simulink model "IEEE30_case"  (R2024b)
settings: Solver=FixedStepAuto  StartTime=0  StopTime=5  FixedStep=1e-7  RelTol=1e-3
values from neighbouring files (symbols this model uses):
  GFL_DFIG_7_C_bus = 0.08    [IEEE30_case_parameters.m]
  GFL_DFIG_7_D_mutual = 2.500000e+3    (= 2500)    [IEEE30_case_parameters.m]
  GFL_DFIG_7_f0 = 60    [IEEE30_case_parameters.m]
  GFL_DFIG_7_gPLLi = 3200    [IEEE30_case_parameters.m]
  GFL_DFIG_7_gPLLp = 650    [IEEE30_case_parameters.m]
  GFL_DFIG_7_H_WT = 0.4    [IEEE30_case_parameters.m]
  GFL_DFIG_7_Hg = 0.8    [IEEE30_case_parameters.m]
  GFL_DFIG_7_Igq_ref = 0    [IEEE30_case_parameters.m]
  GFL_DFIG_7_Ird_ref = 704.45696    [IEEE30_case_parameters.m]
  GFL_DFIG_7_KI_V = -300000    [IEEE30_case_parameters.m]
  GFL_DFIG_7_KP_V = -1000    [IEEE30_case_parameters.m]
  GFL_DFIG_7_Ksh = 1.254300e+4    (= 12543)    [IEEE30_case_parameters.m]
  GFL_DFIG_7_Lg = 0.000483    [IEEE30_case_parameters.m]
  GFL_DFIG_7_Lm_pu = 4    [IEEE30_case_parameters.m]
  GFL_DFIG_7_N = 100    [IEEE30_case_parameters.m]
  GFL_DFIG_7_p = 2    [IEEE30_case_parameters.m]
  GFL_DFIG_7_Pitch = 0    [IEEE30_case_parameters.m]
  GFL_DFIG_7_R = 44    [IEEE30_case_parameters.m]
  GFL_DFIG_7_Rg = 2.000000e-5    (= 2e-05)    [IEEE30_case_parameters.m]
  GFL_DFIG_7_rho = 1.225    [IEEE30_case_parameters.m]
  GFL_DFIG_7_rPLLi = 4500    [IEEE30_case_parameters.m]
  GFL_DFIG_7_rPLLp = 620    [IEEE30_case_parameters.m]
  GFL_DFIG_7_Rs_pu = 0.011    [IEEE30_case_parameters.m]
  GFL_DFIG_7_Sbase = 2.000000e+6    (= 2000000)    [IEEE30_case_parameters.m]
  GFL_DFIG_7_ugq_ref = 0    [IEEE30_case_parameters.m]
  GFL_DFIG_7_usd_ref = 0    [IEEE30_case_parameters.m]
  GFL_DFIG_7_Vbase = 690    [IEEE30_case_parameters.m]
  GFL_DFIG_7_Vdc_ref = 1200    [IEEE30_case_parameters.m]
  GFL_DFIG_7_wind = 12    [IEEE30_case_parameters.m]
  GFL_DFIG_7_wm_ref = 518.184209    [IEEE30_case_parameters.m]
  SG_D_13_D = 0.01056    [IEEE30_case_parameters.m]
  SG_D_13_EnableSaturation = 0    [IEEE30_case_parameters.m]
  SG_D_13_f0 = 60    [IEEE30_case_parameters.m]
  SG_D_13_H = 7.5    [IEEE30_case_parameters.m]
  SG_D_13_K_A = 20    [IEEE30_case_parameters.m]
  SG_D_13_K_E = 1.000000e+1    (= 10)    [IEEE30_case_parameters.m]
  SG_D_13_K_F = 2.363    [IEEE30_case_parameters.m]
  SG_D_13_K_s = 0.5    [IEEE30_case_parameters.m]
  SG_D_13_R_a = 0.001088    [IEEE30_case_parameters.m]
  SG_D_13_S_A = 1    [IEEE30_case_parameters.m]
  SG_D_13_S_B = 0.103    [IEEE30_case_parameters.m]
  SG_D_13_S_N = 10.659857    [IEEE30_case_parameters.m]
  SG_D_13_SpeedPara = 200    [IEEE30_case_parameters.m]
  SG_D_13_T_0 = 0.370163    [IEEE30_case_parameters.m]
  SG_D_13_T_1 = 0.3    [IEEE30_case_parameters.m]
  SG_D_13_T_2 = 0.05    [IEEE30_case_parameters.m]
  SG_D_13_T_3 = 0.02    [IEEE30_case_parameters.m]
  SG_D_13_T_4 = 0.005    [IEEE30_case_parameters.m]
  SG_D_13_T_A = 0.02    [IEEE30_case_parameters.m]
  SG_D_13_T_dd = 8.000000e+0    (= 8)    [IEEE30_case_parameters.m]
  SG_D_13_T_ddd = 0.04    [IEEE30_case_parameters.m]
  SG_D_13_T_E = 0.314    [IEEE30_case_parameters.m]
  SG_D_13_T_F = 0.35    [IEEE30_case_parameters.m]
  SG_D_13_T_qd = 0.8    [IEEE30_case_parameters.m]
  SG_D_13_T_qdd = 0.02    [IEEE30_case_parameters.m]
  SG_D_13_T_speed = 0.1    [IEEE30_case_parameters.m]
  SG_D_13_T_w = 0.5    [IEEE30_case_parameters.m]
  SG_D_13_V_ref = 1.696619    [IEEE30_case_parameters.m]
  SG_D_13_w_ref = 376.991118    [IEEE30_case_parameters.m]
  SG_D_13_x_d = 1.9    [IEEE30_case_parameters.m]
  SG_D_13_x_dd = 0.302    [IEEE30_case_parameters.m]
  SG_D_13_x_ddd = 0.204    [IEEE30_case_parameters.m]
  SG_D_13_x_l = 0.05    [IEEE30_case_parameters.m]
  SG_D_13_x_q = 1.3    [IEEE30_case_parameters.m]
  SG_D_13_x_qd = 0.5    [IEEE30_case_parameters.m]
  SG_D_13_x_qdd = 0.3    [IEEE30_case_parameters.m]
  SG_D_1_D = 0.01056    [IEEE30_case_parameters.m]
  SG_D_1_EnableSaturation = 0    [IEEE30_case_parameters.m]
  SG_D_1_f0 = 60    [IEEE30_case_parameters.m]
  SG_D_1_H = 7.5    [IEEE30_case_parameters.m]
  SG_D_1_K_A = 20    [IEEE30_case_parameters.m]
  SG_D_1_K_E = 1.000000e+1    (= 10)    [IEEE30_case_parameters.m]
  SG_D_1_K_F = 2.363    [IEEE30_case_parameters.m]
  SG_D_1_K_s = 0.5    [IEEE30_case_parameters.m]
  SG_D_1_R_a = 0.001088    [IEEE30_case_parameters.m]
  SG_D_1_S_A = 1    [IEEE30_case_parameters.m]
  SG_D_1_S_B = 0.103    [IEEE30_case_parameters.m]
  SG_D_1_S_N = 10.659857    [IEEE30_case_parameters.m]
  SG_D_1_SpeedPara = 200    [IEEE30_case_parameters.m]
  SG_D_1_T_0 = 0.259812    [IEEE30_case_parameters.m]
  SG_D_1_T_1 = 0.3    [IEEE30_case_parameters.m]
  SG_D_1_T_2 = 0.05    [IEEE30_case_parameters.m]
  SG_D_1_T_3 = 0.02    [IEEE30_case_parameters.m]
  SG_D_1_T_4 = 0.005    [IEEE30_case_parameters.m]
  SG_D_1_T_A = 0.02    [IEEE30_case_parameters.m]
  SG_D_1_T_dd = 8.000000e+0    (= 8)    [IEEE30_case_parameters.m]
  SG_D_1_T_ddd = 0.04    [IEEE30_case_parameters.m]
  SG_D_1_T_E = 0.314    [IEEE30_case_parameters.m]
  SG_D_1_T_F = 0.35    [IEEE30_case_parameters.m]
  SG_D_1_T_qd = 0.8    [IEEE30_case_parameters.m]
  SG_D_1_T_qdd = 0.02    [IEEE30_case_parameters.m]
  SG_D_1_T_speed = 0.1    [IEEE30_case_parameters.m]
  SG_D_1_T_w = 0.5    [IEEE30_case_parameters.m]
  SG_D_1_V_ref = 1.544107    [IEEE30_case_parameters.m]
  SG_D_1_w_ref = 376.991118    [IEEE30_case_parameters.m]
  SG_D_1_x_d = 1.9    [IEEE30_case_parameters.m]
  SG_D_1_x_dd = 0.302    [IEEE30_case_parameters.m]
  SG_D_1_x_ddd = 0.204    [IEEE30_case_parameters.m]
  SG_D_1_x_l = 0.05    [IEEE30_case_parameters.m]
  SG_D_1_x_q = 1.3    [IEEE30_case_parameters.m]
  SG_D_1_x_qd = 0.5    [IEEE30_case_parameters.m]
  SG_D_1_x_qdd = 0.3    [IEEE30_case_parameters.m]
  SG_D_22_D = 0.01056    [IEEE30_case_parameters.m]
  SG_D_22_EnableSaturation = 0    [IEEE30_case_parameters.m]
  SG_D_22_f0 = 60    [IEEE30_case_parameters.m]
  SG_D_22_H = 7.5    [IEEE30_case_parameters.m]
  SG_D_22_K_A = 20    [IEEE30_case_parameters.m]
  SG_D_22_K_E = 1.000000e+1    (= 10)    [IEEE30_case_parameters.m]
  SG_D_22_K_F = 2.363    [IEEE30_case_parameters.m]
  SG_D_22_K_s = 0.5    [IEEE30_case_parameters.m]
  SG_D_22_R_a = 0.001088    [IEEE30_case_parameters.m]
  SG_D_22_S_A = 1    [IEEE30_case_parameters.m]
  SG_D_22_S_B = 0.103    [IEEE30_case_parameters.m]
  SG_D_22_S_N = 10.659857    [IEEE30_case_parameters.m]
  SG_D_22_SpeedPara = 200    [IEEE30_case_parameters.m]
  SG_D_22_T_0 = 0.216121    [IEEE30_case_parameters.m]
  SG_D_22_T_1 = 0.3    [IEEE30_case_parameters.m]
  SG_D_22_T_2 = 0.05    [IEEE30_case_parameters.m]
  SG_D_22_T_3 = 0.02    [IEEE30_case_parameters.m]
  SG_D_22_T_4 = 0.005    [IEEE30_case_parameters.m]
  ... (+126 more)
(part 12 of 27)

== system IEEE30_case/GFL_DFIG_7/d_Phi_gb_GFL_DFIG_7_block ==
  note: d_Phi_gb_GFL_DFIG_7 in IEEE30_case
      | $-4\,\mathrm{Lg}\,{f_{0}}^2\,\pi ^2\,\left(i_{\mathrm{gd},\mathrm{GFL},\mathrm{DFIG},7}-\frac{0.666666666666667\,\Phi _{\mathrm{gc},\mathrm{GFL},\mathrm{DFIG},7}-0.666666666666667\,\mathrm{KP}_{V}\,\left(V_{\mathrm{dc},\mathrm{GFL},\mathrm{DFIG},7}-\mathrm{Vdc}_{\mathrm{ref}}\right)}{\mathrm{Vbase}}\right)$
      | Automatically generated on 2025-11-01 18:34:05 .
  State_i_gd_GFL_DFIG_7_640f4 : Inport
  State_V_dc_GFL_DFIG_7_6d222 : Inport  Port=2
  State_Phi_gc_GFL_DFIG_7_b7107 : Inport  Port=3
  Add_6bffb : Sum
  Add_b5257 : Sum
  Add_b8cf5 : Sum
  Constant_-1_6b980 : Constant  Value=-1
  Constant_-1_cf33c : Constant  Value=-1
  Constant_0.666666666666667_f141c : Constant  Value=0.666666666666667
  Constant_2.0_6b877 : Constant  Value=2.0
  Constant_2.0_f717f : Constant  Value=2.0
  Constant_4.0_b6ef0 : Constant  Value=4.0
  Constant_KP_V_1bd51 : Constant  Value=KP_V
  Constant_Lg_6a87d : Constant  Value=Lg
  Constant_Vbase_73b54 : Constant  Value=Vbase
  Constant_Vdc_ref_f08aa : Constant  Value=Vdc_ref
  Constant_f0_de8e9 : Constant  Value=f0
  Constant_pi_e3308 : Constant  Value=pi
  Divide_9162a : Product  Inputs=*/
  Power_585c5 : Math  Operator=pow
  Power_96685 : Math  Operator=pow
  Product_0199e : Product
  Product_1d506 : Product
  Product_26373 : Product
  Product_b2acb : Product
  Product_c600a : Product
  Product_cfa46 : Product
  Product_d4dd0 : Product
  Product_f39e3 : Product
  Blockout_d_Phi_gb_GFL_DFIG_7_12bfd : Outport
  wires:
  Constant_-1_6b980/1 -> Product_d4dd0/1
  Constant_Vdc_ref_f08aa/1 -> Add_b8cf5/2
  Constant_pi_e3308/1 -> Power_96685/1
  Constant_Vbase_73b54/1 -> Divide_9162a/2
  Add_b8cf5/1 -> Product_c600a/2
  State_V_dc_GFL_DFIG_7_6d222/1 -> Product_d4dd0/2
  Product_d4dd0/1 -> Add_b8cf5/1
  State_i_gd_GFL_DFIG_7_640f4/1 -> Product_1d506/2
  Constant_KP_V_1bd51/1 -> Product_c600a/1
  Constant_2.0_f717f/1 -> Power_96685/2
  Product_c600a/1 -> Add_b5257/1
  State_Phi_gc_GFL_DFIG_7_b7107/1 -> Add_b5257/2
  Constant_4.0_b6ef0/1 -> Product_26373/1
  Power_96685/1 -> Product_26373/2
  Constant_0.666666666666667_f141c/1 -> Product_cfa46/1
  Product_0199e/1 -> Product_b2acb/1
  Add_b5257/1 -> Product_cfa46/2
  Product_26373/1 -> Product_f39e3/1
  Constant_f0_de8e9/1 -> Power_585c5/1
  Constant_Lg_6a87d/1 -> Product_f39e3/2
  Constant_2.0_6b877/1 -> Power_585c5/2
  Constant_-1_cf33c/1 -> Product_1d506/1
  Product_cfa46/1 -> Divide_9162a/1
  Product_f39e3/1 -> Product_0199e/1
  Power_585c5/1 -> Product_0199e/2
  Product_1d506/1 -> Add_6bffb/1
  Divide_9162a/1 -> Add_6bffb/2
  Add_6bffb/1 -> Product_b2acb/2
  Product_b2acb/1 -> Blockout_d_Phi_gb_GFL_DFIG_7_12bfd/1

== system IEEE30_case/GFL_DFIG_7/d_Phi_gc_GFL_DFIG_7_block ==
  note: d_Phi_gc_GFL_DFIG_7 in IEEE30_case
      | $-\mathrm{KI}_{V}\,\left(V_{\mathrm{dc},\mathrm{GFL},\mathrm{DFIG},7}-\mathrm{Vdc}_{\mathrm{ref}}\right)$
      | Automatically generated on 2025-11-01 18:34:03 .
  State_V_dc_GFL_DFIG_7_30c65 : Inport
  Add_e8db4 : Sum
  Constant_-1_5cb89 : Constant  Value=-1
  Constant_KI_V_c5ac4 : Constant  Value=KI_V
  Constant_Vdc_ref_57ce9 : Constant  Value=Vdc_ref
  Product_3b29a : Product
  Product_b79c6 : Product
  Blockout_d_Phi_gc_GFL_DFIG_7_e7a32 : Outport
  wires:
  Constant_-1_5cb89/1 -> Product_3b29a/1
  State_V_dc_GFL_DFIG_7_30c65/1 -> Product_3b29a/2
  Product_3b29a/1 -> Add_e8db4/1
  Product_b79c6/1 -> Blockout_d_Phi_gc_GFL_DFIG_7_e7a32/1
  Constant_Vdc_ref_57ce9/1 -> Add_e8db4/2
  Constant_KI_V_c5ac4/1 -> Product_b79c6/1
  Add_e8db4/1 -> Product_b79c6/2

== system IEEE30_case/GFL_DFIG_7/d_Phi_ra_GFL_DFIG_7_block ==
  note: d_Phi_ra_GFL_DFIG_7 in IEEE30_case
      | $\frac{121.601990049751\,\pi \,{\mathrm{Rs}_{\mathrm{pu}}}^2\,{\mathrm{Vbase}}^2\,f_{0}\,\left(\mathrm{Ird}_{\mathrm{ref}}-\frac{100.497512437811\,\pi \,\Psi _{\mathrm{dr},\mathrm{GFL},\mathrm{DFIG},7}\,\mathrm{Sbase}\,f_{0}}{\mathrm{Lm}_{\mathrm{pu}}\,{\mathrm{Vbase}}^2}+\frac{99.502487562189\,\pi \,\Psi _{\mathrm{ds},\mathrm{GFL},\mathrm{DFIG},7}\,\mathrm{Sbase}\,f_{0}}{\mathrm{Lm}_{\mathrm{pu}}\,{\mathrm{Vbase}}^2}\right)}{\mathrm{Lm}_{\mathrm{pu}}\,\mathrm{Sbase}}$
      | Automatically generated on 2025-11-01 18:33:11 .
  State_Psi_dr_GFL_DFIG_7_3e6d6 : Inport
  State_Psi_ds_GFL_DFIG_7_9adb5 : Inport  Port=2
  Add_f4b53 : Sum
  Constant_100.497512437811_3d4e5 : Constant  Value=100.497512437811
  Constant_121.601990049751_8103e : Constant  Value=121.601990049751
  Constant_2.0_5d4a4 : Constant  Value=2.0
  Constant_2.0_83c42 : Constant  Value=2.0
  Constant_2.0_893ba : Constant  Value=2.0
  Constant_2.0_ddf2f : Constant  Value=2.0
  Constant_99.502487562189_4b56a : Constant  Value=99.502487562189
  Constant_Ird_ref_83d74 : Constant  Value=Ird_ref
  Constant_Lm_pu_11795 : Constant  Value=Lm_pu
  Constant_Lm_pu_a81e2 : Constant  Value=Lm_pu
  Constant_Lm_pu_dbc9c : Constant  Value=Lm_pu
  Constant_Rs_pu_66a36 : Constant  Value=Rs_pu
  Constant_Sbase_aa7f6 : Constant  Value=Sbase
  Constant_Sbase_e8890 : Constant  Value=Sbase
  Constant_Sbase_efa73 : Constant  Value=Sbase
  Constant_Vbase_4a93a : Constant  Value=Vbase
  Constant_Vbase_63b23 : Constant  Value=Vbase
  Constant_Vbase_ff58f : Constant  Value=Vbase
  Constant_f0_6d6a3 : Constant  Value=f0
  Constant_f0_798e9 : Constant  Value=f0
  Constant_f0_b0c51 : Constant  Value=f0
  Constant_pi_37fdb : Constant  Value=pi
  Constant_pi_c8d94 : Constant  Value=pi
  Constant_pi_e7969 : Constant  Value=pi
  Divide_0905f : Product  Inputs=*/
  Divide_383a0 : Product  Inputs=*/
  Divide_99316 : Product  Inputs=*/
  Power_35857 : Math  Operator=pow
  Power_5b5c9 : Math  Operator=pow
  Power_dc40c : Math  Operator=pow
  Power_df89a : Math  Operator=pow
  Product_081b4 : Product
  Product_09a91 : Product
  Product_12e3f : Product
  Product_15670 : Product
  Product_186d4 : Product
  Product_26318 : Product
  Product_38ada : Product
  Product_3f361 : Product
  Product_5c4f4 : Product
  Product_684e9 : Product
  Product_8995b : Product
  Product_96f38 : Product
  Product_aa582 : Product
  Product_b7735 : Product
  Product_d9359 : Product
  Product_d9bcd : Product
  Subtract_8a7b5 : Sum  Inputs=+-
  Blockout_d_Phi_ra_GFL_DFIG_7_b9bb2 : Outport
  wires:
  Constant_Sbase_efa73/1 -> Product_12e3f/2
  Constant_100.497512437811_3d4e5/1 -> Product_38ada/1
  Constant_Vbase_ff58f/1 -> Power_5b5c9/1
  Product_96f38/1 -> Product_15670/1
  Constant_2.0_83c42/1 -> Power_35857/2
  Constant_pi_37fdb/1 -> Product_38ada/2
  State_Psi_dr_GFL_DFIG_7_3e6d6/1 -> Product_96f38/2
  Product_d9bcd/1 -> Product_5c4f4/1
  Product_38ada/1 -> Product_96f38/1
  Constant_99.502487562189_4b56a/1 -> Product_26318/1
  Product_5c4f4/1 -> Product_186d4/1
  Constant_pi_c8d94/1 -> Product_26318/2
  Constant_Vbase_63b23/1 -> Power_dc40c/1
  Constant_Sbase_aa7f6/1 -> Product_15670/2
  Constant_Vbase_4a93a/1 -> Power_df89a/1
  Constant_2.0_893ba/1 -> Power_df89a/2
  Product_26318/1 -> Product_aa582/1
  State_Psi_ds_GFL_DFIG_7_9adb5/1 -> Product_aa582/2
  Constant_Sbase_e8890/1 -> Product_8995b/2
  Constant_Rs_pu_66a36/1 -> Power_35857/1
  Constant_121.601990049751_8103e/1 -> Product_d9bcd/1
  Constant_pi_e7969/1 -> Product_d9bcd/2
  Product_8995b/1 -> Divide_99316/2
  Product_15670/1 -> Product_081b4/1
  Product_3f361/1 -> Product_b7735/1
  Constant_f0_798e9/1 -> Product_081b4/2
  Product_b7735/1 -> Divide_99316/1
  Constant_Lm_pu_a81e2/1 -> Product_684e9/1
  Power_df89a/1 -> Product_684e9/2
  Product_aa582/1 -> Product_12e3f/1
  Constant_2.0_5d4a4/1 -> Power_5b5c9/2
  Power_35857/1 -> Product_5c4f4/2
  Constant_2.0_ddf2f/1 -> Power_dc40c/2
  Product_081b4/1 -> Divide_0905f/1
  Product_684e9/1 -> Divide_0905f/2
  Product_12e3f/1 -> Product_09a91/1
  Divide_383a0/1 -> Add_f4b53/2
  Constant_f0_6d6a3/1 -> Product_09a91/2
  Constant_Lm_pu_11795/1 -> Product_d9359/1
  Power_5b5c9/1 -> Product_d9359/2
  Power_dc40c/1 -> Product_186d4/2
  Constant_Ird_ref_83d74/1 -> Subtract_8a7b5/1
  Divide_0905f/1 -> Subtract_8a7b5/2
  Product_09a91/1 -> Divide_383a0/1
  Product_d9359/1 -> Divide_383a0/2
  Product_186d4/1 -> Product_3f361/1
  Constant_f0_b0c51/1 -> Product_3f361/2
  Subtract_8a7b5/1 -> Add_f4b53/1
  Add_f4b53/1 -> Product_b7735/2
  Constant_Lm_pu_dbc9c/1 -> Product_8995b/1
  Divide_99316/1 -> Blockout_d_Phi_ra_GFL_DFIG_7_b9bb2/1

== system IEEE30_case/GFL_DFIG_7/d_Phi_rb_GFL_DFIG_7_block ==
  note: d_Phi_rb_GFL_DFIG_7 in IEEE30_case
      | $-\frac{121.601990049751\,\pi \,{\mathrm{Rs}_{\mathrm{pu}}}^2\,{\mathrm{Vbase}}^2\,f_{0}\,\left(\frac{0.673333333333333\,\Phi _{\mathrm{rc},\mathrm{GFL},\mathrm{DFIG},7}-\frac{10.773333333333328\,\mathrm{Sbase}\,p\,\left(w_{m,\mathrm{GFL},\mathrm{DFIG},7}-\mathrm{wm}_{\mathrm{ref}}\right)}{{f_{0}}^2\,\pi ^2}}{p\,\sqrt{{\Psi _{\mathrm{ds},\mathrm{GFL},\mathrm{DFIG},7}}^2+{\Psi _{\mathrm{qs},\mathrm{GFL},\mathrm{DFIG},7}}^2}}+\frac{100.497512437811\,\pi \,\Psi _{\mathrm{qr},\mathrm{GFL},\mathrm{DFIG},7}\,\mathrm{Sbase}\,f_{0}}{\mathrm{Lm}_{\mathrm{pu}}\,{\mathrm{Vbase}}^2}-\frac{99.502487562189\,\pi \,\Psi _{\mathrm{qs},\mathrm{GFL},\mathrm{DFIG},7}\,\mathrm{Sbase}\,f_{0}}{\mathrm{Lm}_{\mathrm{pu}}\,{\mathrm{Vbase}}^2}\right)}{\mathrm{Lm}_{\mathrm{pu}}\,\mathrm{Sbase}}$
      | Automatically generated on 2025-11-01 18:33:17 .
  State_Phi_rc_GFL_DFIG_7_bc2c9 : Inport
  State_w_m_GFL_DFIG_7_5425d : Inport  Port=2
  State_Psi_ds_GFL_DFIG_7_7a16b : Inport  Port=3
  State_Psi_qs_GFL_DFIG_7_57503 : Inport  Port=4
  State_Psi_qr_GFL_DFIG_7_e4388 : Inport  Port=5
  State_Psi_qs_GFL_DFIG_7_e35cc : Inport  Port=6
  Add_8c335 : Sum
  Add_8e695 : Sum
  Add_9cf97 : Sum
  Add_d9e26 : Sum
  Constant_-0.673333333333333_fade5 : Constant  Value=-0.673333333333333
  Constant_-1_8d982 : Constant  Value=-1
  Constant_100.497512437811_2b07e : Constant  Value=100.497512437811
  Constant_121.601990049751_b651a : Constant  Value=121.601990049751
  Constant_16.0_b18cb : Constant  Value=16.0
  Constant_2.0_154d8 : Constant  Value=2.0
  Constant_2.0_24e66 : Constant  Value=2.0
  Constant_2.0_2b9f3 : Constant  Value=2.0
  Constant_2.0_3bf41 : Constant  Value=2.0
  Constant_2.0_59165 : Constant  Value=2.0
  Constant_2.0_c1799 : Constant  Value=2.0
  Constant_2.0_c26f1 : Constant  Value=2.0
  Constant_2.0_f645a : Constant  Value=2.0
  Constant_99.502487562189_3da1b : Constant  Value=99.502487562189
  Constant_Lm_pu_c3cbe : Constant  Value=Lm_pu
  Constant_Lm_pu_c51f7 : Constant  Value=Lm_pu
  Constant_Lm_pu_fef3e : Constant  Value=Lm_pu
  Constant_Rs_pu_8b800 : Constant  Value=Rs_pu
  Constant_Sbase_1934d : Constant  Value=Sbase
  Constant_Sbase_2886b : Constant  Value=Sbase
  Constant_Sbase_44824 : Constant  Value=Sbase
  Constant_Sbase_acc82 : Constant  Value=Sbase
  Constant_Vbase_057c8 : Constant  Value=Vbase
  Constant_Vbase_33be2 : Constant  Value=Vbase
  Constant_Vbase_c886f : Constant  Value=Vbase
  Constant_f0_37fb8 : Constant  Value=f0
  Constant_f0_64fd6 : Constant  Value=f0
  Constant_f0_d2cee : Constant  Value=f0
  Constant_f0_e037e : Constant  Value=f0
  Constant_p_9dc95 : Constant  Value=p
  Constant_p_ae0c5 : Constant  Value=p
  Constant_pi_2d1cb : Constant  Value=pi
  Constant_pi_5eceb : Constant  Value=pi
  Constant_pi_5ef27 : Constant  Value=pi
  Constant_pi_b22d2 : Constant  Value=pi
  Constant_wm_ref_5b7e7 : Constant  Value=wm_ref
  Divide_0adfc : Product  Inputs=*/
  Divide_2d540 : Product  Inputs=*/
  Divide_6bab9 : Product  Inputs=*/
  Divide_9109e : Product  Inputs=*/
  Divide_a367a : Product  Inputs=*/
  MathFunc_sqrt_aa524 : Sqrt
  Power_02213 : Math  Operator=pow
  Power_34a99 : Math  Operator=pow
  Power_4517e : Math  Operator=pow
  Power_abf73 : Math  Operator=pow
  Power_c1057 : Math  Operator=pow
  Power_c8651 : Math  Operator=pow
  Power_d591f : Math  Operator=pow
  Power_f198e : Math  Operator=pow
  Product_105da : Product
  Product_147e3 : Product
  Product_24720 : Product
  Product_307a1 : Product
  Product_3f565 : Product
  Product_436c9 : Product
  Product_4cf24 : Product
  Product_5f731 : Product
  Product_6572c : Product
  Product_6d301 : Product
  Product_6da22 : Product
  Product_6ecc6 : Product
  Product_96586 : Product
  Product_99f2d : Product
  Product_a3501 : Product
  Product_ba56f : Product
  Product_c0d1a : Product
  Product_c2194 : Product
  Product_c2604 : Product
  Product_d5eee : Product
  Product_dfcd2 : Product
  Product_e7fe8 : Product
  Product_eb59e : Product
  Subtract_2b91f : Sum  Inputs=+-
  Blockout_d_Phi_rb_GFL_DFIG_7_7ae6c : Outport
  wires:
  Constant_Sbase_acc82/1 -> Product_96586/2
  Constant_16.0_b18cb/1 -> Product_dfcd2/1
  Constant_p_9dc95/1 -> Product_6da22/2
  Product_5f731/1 -> Divide_0adfc/1
  State_Psi_qr_GFL_DFIG_7_e4388/1 -> Product_a3501/2
  Constant_Sbase_2886b/1 -> Product_dfcd2/2
  Constant_100.497512437811_2b07e/1 -> Product_147e3/1
  Constant_wm_ref_5b7e7/1 -> Add_9cf97/2
  Constant_Lm_pu_c51f7/1 -> Product_99f2d/1
  Constant_-1_8d982/1 -> Product_c2604/1
  Product_dfcd2/1 -> Product_6da22/1
  State_w_m_GFL_DFIG_7_5425d/1 -> Product_c2604/2
  Product_99f2d/1 -> Divide_2d540/2
  Product_c2604/1 -> Add_9cf97/1
  Constant_pi_b22d2/1 -> Power_4517e/1
  Constant_2.0_c1799/1 -> Power_4517e/2
  Product_c2194/1 -> Product_105da/1
  Constant_f0_64fd6/1 -> Power_f198e/1
  Constant_2.0_2b9f3/1 -> Power_f198e/2
  Product_147e3/1 -> Product_a3501/1
  Product_6da22/1 -> Product_6ecc6/1
  Add_9cf97/1 -> Product_6ecc6/2
  Power_4517e/1 -> Product_eb59e/1
  Product_105da/1 -> Product_6572c/1
  Product_3f565/1 -> Product_ba56f/1
  Power_f198e/1 -> Product_eb59e/2
  State_Psi_ds_GFL_DFIG_7_7a16b/1 -> Power_34a99/1
  Constant_2.0_c26f1/1 -> Power_34a99/2
  State_Psi_qs_GFL_DFIG_7_57503/1 -> Power_02213/1
  Constant_2.0_f645a/1 -> Power_02213/2
  Constant_pi_2d1cb/1 -> Product_147e3/2
  Product_a3501/1 -> Product_96586/1
  Product_6ecc6/1 -> Divide_9109e/1
  Product_eb59e/1 -> Divide_9109e/2
  Constant_pi_5eceb/1 -> Product_3f565/2
  Power_34a99/1 -> Add_8e695/1
  Constant_2.0_3bf41/1 -> Power_c8651/2
  Power_02213/1 -> Add_8e695/2
  Power_abf73/1 -> Product_ba56f/2
  Constant_99.502487562189_3da1b/1 -> Product_d5eee/1
  Constant_pi_5ef27/1 -> Product_d5eee/2
  State_Phi_rc_GFL_DFIG_7_bc2c9/1 -> Add_d9e26/1
  Product_96586/1 -> Product_6d301/1
  Divide_9109e/1 -> Add_d9e26/2
  Constant_Vbase_33be2/1 -> Power_d591f/1
  Add_8e695/1 -> MathFunc_sqrt_aa524/1
  Constant_Vbase_057c8/1 -> Power_c1057/1
  Constant_2.0_154d8/1 -> Power_c1057/2
  Product_d5eee/1 -> Product_c2194/1
  State_Psi_qs_GFL_DFIG_7_e35cc/1 -> Product_c2194/2
  Constant_121.601990049751_b651a/1 -> Product_3f565/1
  Constant_Sbase_1934d/1 -> Product_105da/2
  Constant_Rs_pu_8b800/1 -> Power_abf73/1
  Product_4cf24/1 -> Divide_6bab9/2
  Constant_2.0_24e66/1 -> Power_abf73/2
  Constant_-0.673333333333333_fade5/1 -> Product_307a1/1
  Add_d9e26/1 -> Product_307a1/2
  Constant_p_ae0c5/1 -> Product_4cf24/1
  MathFunc_sqrt_aa524/1 -> Product_4cf24/2
  Constant_f0_d2cee/1 -> Product_6d301/2
  Power_c1057/1 -> Product_99f2d/2
  Constant_Vbase_c886f/1 -> Power_c8651/1
  Constant_2.0_59165/1 -> Power_d591f/2
  Product_307a1/1 -> Divide_6bab9/1
  Product_6d301/1 -> Divide_2d540/1
  Constant_f0_e037e/1 -> Product_6572c/2
  Constant_Lm_pu_c3cbe/1 -> Product_c0d1a/1
  Power_c8651/1 -> Product_c0d1a/2
  Product_ba56f/1 -> Product_436c9/1
  Power_d591f/1 -> Product_436c9/2
  Divide_6bab9/1 -> Subtract_2b91f/1
  Divide_2d540/1 -> Subtract_2b91f/2
  Product_6572c/1 -> Divide_a367a/1
  Product_c0d1a/1 -> Divide_a367a/2
  Product_436c9/1 -> Product_24720/1
  Constant_f0_37fb8/1 -> Product_24720/2
  Subtract_2b91f/1 -> Add_8c335/1
  Divide_a367a/1 -> Add_8c335/2
  Product_24720/1 -> Product_5f731/1
  Add_8c335/1 -> Product_5f731/2
  Constant_Lm_pu_fef3e/1 -> Product_e7fe8/1
  Constant_Sbase_44824/1 -> Product_e7fe8/2
  Product_e7fe8/1 -> Divide_0adfc/2
  Divide_0adfc/1 -> Blockout_d_Phi_rb_GFL_DFIG_7_7ae6c/1

== system IEEE30_case/GFL_DFIG_7/d_Phi_rc_GFL_DFIG_7_block ==
  note: d_Phi_rc_GFL_DFIG_7 in IEEE30_case
      | $-\frac{128\,\mathrm{Sbase}\,p\,\left(w_{m,\mathrm{GFL},\mathrm{DFIG},7}-\mathrm{wm}_{\mathrm{ref}}\right)}{\mathrm{Hg}\,{f_{0}}^2\,\pi ^2}$
      | Automatically generated on 2025-11-01 18:33:13 .
  State_w_m_GFL_DFIG_7_b5946 : Inport
  Add_033cf : Sum
  Constant_-1_a203c : Constant  Value=-1
  Constant_128.0_a6df2 : Constant  Value=128.0
  Constant_2.0_1c071 : Constant  Value=2.0
  Constant_2.0_c935a : Constant  Value=2.0
  Constant_Hg_01f24 : Constant  Value=Hg
  Constant_Sbase_867f4 : Constant  Value=Sbase
  Constant_f0_a5d67 : Constant  Value=f0
  Constant_p_14ae6 : Constant  Value=p
  Constant_pi_9f808 : Constant  Value=pi
  Constant_wm_ref_67022 : Constant  Value=wm_ref
  Divide_7ffd1 : Product  Inputs=*/
  Power_0f740 : Math  Operator=pow
  Power_99261 : Math  Operator=pow
  Product_167f3 : Product
  Product_23ecd : Product
  Product_336df : Product
  Product_343c6 : Product
  Product_bafc2 : Product
  Product_d8355 : Product
  Blockout_d_Phi_rc_GFL_DFIG_7_aa447 : Outport
  wires:
  Constant_p_14ae6/1 -> Product_167f3/2
  Constant_128.0_a6df2/1 -> Product_343c6/1
  State_w_m_GFL_DFIG_7_b5946/1 -> Product_23ecd/2
  Constant_Sbase_867f4/1 -> Product_343c6/2
  Product_bafc2/1 -> Divide_7ffd1/1
  Constant_2.0_c935a/1 -> Power_99261/2
  Constant_-1_a203c/1 -> Product_23ecd/1
  Constant_Hg_01f24/1 -> Product_336df/2
  Product_23ecd/1 -> Add_033cf/1
  Constant_pi_9f808/1 -> Power_99261/1
  Product_343c6/1 -> Product_167f3/1
  Constant_wm_ref_67022/1 -> Add_033cf/2
  Power_99261/1 -> Product_336df/1
  Constant_f0_a5d67/1 -> Power_0f740/1
  Add_033cf/1 -> Product_bafc2/2
  Constant_2.0_1c071/1 -> Power_0f740/2
  Product_167f3/1 -> Product_bafc2/1
  Product_336df/1 -> Product_d8355/1
  Power_0f740/1 -> Product_d8355/2
  Product_d8355/1 -> Divide_7ffd1/2
  Divide_7ffd1/1 -> Blockout_d_Phi_rc_GFL_DFIG_7_aa447/1

== system IEEE30_case/GFL_DFIG_7/d_Phipllg_GFL_DFIG_7_block ==
  note: d_Phipllg_GFL_DFIG_7 in IEEE30_case
      | $-\mathrm{gPLLi}\,\left(\mathrm{ugq}_{\mathrm{ref}}+v_{q,\mathrm{GFL},\mathrm{DFIG},7}\,\cos\left(\theta _{\mathrm{pllg},\mathrm{GFL},\mathrm{DFIG},7}\right)+v_{d,\mathrm{GFL},\mathrm{DFIG},7}\,\sin\left(\theta _{\mathrm{pllg},\mathrm{GFL},\mathrm{DFIG},7}\right)\right)$
      | Automatically generated on 2025-11-01 18:34:08 .
  Input_v_d_GFL_DFIG_7_9bb07 : Inport
  State_theta_pllg_GFL_DFIG_7_d7c88 : Inport  Port=2
  Input_v_q_GFL_DFIG_7_4b381 : Inport  Port=3
  State_theta_pllg_GFL_DFIG_7_1f5b3 : Inport  Port=4
  Constant_-1_a8696 : Constant  Value=-1
  Constant_gPLLi_864bf : Constant  Value=gPLLi
  Constant_ugq_ref_056c0 : Constant  Value=ugq_ref
  MathFunc_cos_0cf31 : Trigonometry  Operator=cos
  MathFunc_sin_67054 : Trigonometry
  Product_3b1f1 : Product
  Product_a74be : Product
  Product_b0d09 : Product
  Product_c8c10 : Product
  Subtract_e5638 : Sum  Inputs=+-
  Subtract_ead05 : Sum  Inputs=+-
  Blockout_d_Phipllg_GFL_DFIG_7_57d75 : Outport
  wires:
  State_theta_pllg_GFL_DFIG_7_d7c88/1 -> MathFunc_sin_67054/1
  MathFunc_sin_67054/1 -> Product_3b1f1/2
  Constant_-1_a8696/1 -> Product_c8c10/1
  Input_v_d_GFL_DFIG_7_9bb07/1 -> Product_3b1f1/1
  Constant_ugq_ref_056c0/1 -> Product_c8c10/2
  State_theta_pllg_GFL_DFIG_7_1f5b3/1 -> MathFunc_cos_0cf31/1
  Product_c8c10/1 -> Subtract_ead05/1
  Product_3b1f1/1 -> Subtract_ead05/2
  Input_v_q_GFL_DFIG_7_4b381/1 -> Product_b0d09/1
  MathFunc_cos_0cf31/1 -> Product_b0d09/2
  Subtract_ead05/1 -> Subtract_e5638/1
  Constant_gPLLi_864bf/1 -> Product_a74be/1
  Product_b0d09/1 -> Subtract_e5638/2
  Subtract_e5638/1 -> Product_a74be/2
  Product_a74be/1 -> Blockout_d_Phipllg_GFL_DFIG_7_57d75/1

== system IEEE30_case/GFL_DFIG_7/d_Phipllr_GFL_DFIG_7_block ==
  note: d_Phipllr_GFL_DFIG_7 in IEEE30_case
      | $-\mathrm{rPLLi}\,\left(\mathrm{usd}_{\mathrm{ref}}+v_{d,\mathrm{GFL},\mathrm{DFIG},7}\,\cos\left(\theta _{\mathrm{pllr},\mathrm{GFL},\mathrm{DFIG},7}\right)-v_{q,\mathrm{GFL},\mathrm{DFIG},7}\,\sin\left(\theta _{\mathrm{pllr},\mathrm{GFL},\mathrm{DFIG},7}\right)\right)$
      | Automatically generated on 2025-11-01 18:34:06 .
  Input_v_d_GFL_DFIG_7_0a8be : Inport
  State_theta_pllr_GFL_DFIG_7_673d7 : Inport  Port=2
  Input_v_q_GFL_DFIG_7_661f6 : Inport  Port=3
  State_theta_pllr_GFL_DFIG_7_c3596 : Inport  Port=4
  Add_40468 : Sum
  Constant_-1_1c422 : Constant  Value=-1
  Constant_rPLLi_c38ff : Constant  Value=rPLLi
  Constant_usd_ref_0a1f3 : Constant  Value=usd_ref
  MathFunc_cos_0c009 : Trigonometry  Operator=cos
  MathFunc_sin_3ef5a : Trigonometry
  Product_1f9ff : Product
  Product_79bb6 : Product
  Product_8a815 : Product
  Product_fc47b : Product
  Subtract_51d6e : Sum  Inputs=+-
  Blockout_d_Phipllr_GFL_DFIG_7_3fa24 : Outport
  wires:
  State_theta_pllr_GFL_DFIG_7_673d7/1 -> MathFunc_cos_0c009/1
  Product_8a815/1 -> Subtract_51d6e/2
  MathFunc_cos_0c009/1 -> Product_8a815/2
  Add_40468/1 -> Product_79bb6/2
  Constant_-1_1c422/1 -> Product_fc47b/1
  Product_fc47b/1 -> Subtract_51d6e/1
  Constant_usd_ref_0a1f3/1 -> Product_fc47b/2
  Input_v_d_GFL_DFIG_7_0a8be/1 -> Product_8a815/1
  State_theta_pllr_GFL_DFIG_7_c3596/1 -> MathFunc_sin_3ef5a/1
  Input_v_q_GFL_DFIG_7_661f6/1 -> Product_1f9ff/1
  MathFunc_sin_3ef5a/1 -> Product_1f9ff/2
  Subtract_51d6e/1 -> Add_40468/1
  Product_1f9ff/1 -> Add_40468/2
  Constant_rPLLi_c38ff/1 -> Product_79bb6/1
  Product_79bb6/1 -> Blockout_d_Phipllr_GFL_DFIG_7_3fa24/1

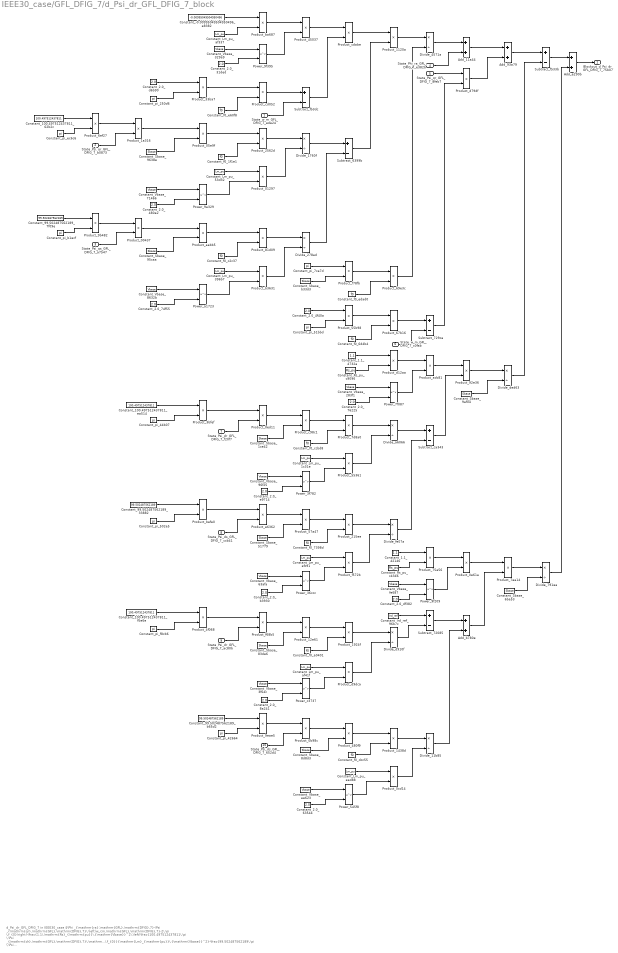
== system IEEE30_case/GFL_DFIG_7/d_Psi_dr_GFL_DFIG_7_block ==
  note: d_Psi_dr_GFL_DFIG_7 in IEEE30_case
      | $\Phi _{\mathrm{ra},\mathrm{GFL},\mathrm{DFIG},7}-\Psi _{\mathrm{qr},\mathrm{GFL},\mathrm{DFIG},7}\,\left(w_{m,\mathrm{GFL},\mathrm{DFIG},7}-2\,\pi \,f_{0}\right)-\frac{1.1\,\mathrm{Rs}_{\mathrm{pu}}\,{\mathrm{Vbase}}^2\,\left(\frac{100.497512437811\,\pi \,\Psi _{\mathrm{dr},\mathrm{GFL},\mathrm{DFIG},7}\,\mathrm{Sbase}\,f_{0}}{\mathrm{Lm}_{\mathrm{pu}}\,{\mathrm{Vbase}}^2}-\frac{99.502487562189\,\pi \,\Psi _{\mathrm{ds},\mathrm{GFL},\mathrm{DFIG},7}\,\mathrm{Sbase}\,f_{0}}{\mathrm{Lm}_{\mathrm{pu}}\,{\mathrm{Vbase}}^2}\right)}{\mathrm{Sbase}}+\frac{1.1\,\mathrm{Rs}_{\mathrm{pu}}\,{\mathrm{Vbase}}^2\,\left(\mathrm{Ird}_{\mathrm{ref}}-\frac{100.497512437811\,\pi \,\Psi _{\mathrm{dr},\mathrm{GFL},\mathrm{DFIG},7}\,\mathrm{Sbase}\,f_{0}}{\mathrm{Lm}_{\mathrm{pu}}\,{\mathrm{Vbase}}^2}+\frac{99.502487562189\,\pi \,\Psi _{\mathrm{ds},\mathrm{GFL},\mathrm{DFIG},7}\,\mathrm{Sbase}\,f_{0}}{\mathrm{Lm}_{\mathrm{pu}}\,{\mathrm{Vbase}}^2}\right)}{\mathrm{Sbase}}+\frac{0.00995049504950496\,\mathrm{Lm}_{\mathrm{pu}}\,{\mathrm{Vbase}}^2\,\left(\frac{100.497512437811\,\pi \,\Psi _{\mathrm{qr},\mathrm{GFL},\mathrm{DFIG},7}\,\mathrm{Sbase}\,f_{0}}{\mathrm{Lm}_{\mathrm{pu}}\,{\mathrm{Vbase}}^2}-\frac{99.502487562189\,\pi \,\Psi _{\mathrm{qs},\mathrm{GFL},\mathrm{DFIG},7}\,\mathrm{Sbase}\,f_{0}}{\mathrm{Lm}_{\mathrm{pu}}\,{\mathrm{Vbase}}^2}\right)\,\left(w_{m,\mathrm{GFL},\mathrm{DFIG},7}-2\,\pi \,f_{0}\right)}{\mathrm{Sbase}\,f_{0}\,\pi }$
      | Automatically generated on 2025-11-01 18:32:46 .
  State_w_m_GFL_DFIG_7_ede24 : Inport
  State_Psi_qr_GFL_DFIG_7_b0873 : Inport  Port=2
  State_Psi_qs_GFL_DFIG_7_a7547 : Inport  Port=3
  State_Phi_ra_GFL_DFIG_7_e382b : Inport  Port=4
  State_Psi_qr_GFL_DFIG_7_8feb7 : Inport  Port=5
  State_w_m_GFL_DFIG_7_c0fab : Inport  Port=6
  State_Psi_dr_GFL_DFIG_7_f20f7 : Inport  Port=7
  State_Psi_ds_GFL_DFIG_7_ccb41 : Inport  Port=8
  State_Psi_dr_GFL_DFIG_7_ac80b : Inport  Port=9
  State_Psi_ds_GFL_DFIG_7_652d4 : Inport  Port=10
  Add_11a44 : Sum
  Add_93a79 : Sum
  Add_b780e : Sum
  Add_e290b : Sum
  Constant_-0.00995049504950496_e8382 : Constant  Value=-0.00995049504950496
  Constant_1.1_42146 : Constant  Value=1.1
  Constant_1.1_4732a : Constant  Value=1.1
  Constant_100.497512437811_62b2c : Constant  Value=100.497512437811
  Constant_100.497512437811_ea514 : Constant  Value=100.497512437811
  Constant_100.497512437811_f5e6e : Constant  Value=100.497512437811
  Constant_2.0_31ded : Constant  Value=2.0
  Constant_2.0_480a2 : Constant  Value=2.0
  Constant_2.0_4f40a : Constant  Value=2.0
  Constant_2.0_63544 : Constant  Value=2.0
  Constant_2.0_74f55 : Constant  Value=2.0
  Constant_2.0_76225 : Constant  Value=2.0
  Constant_2.0_8a241 : Constant  Value=2.0
  Constant_2.0_b3930 : Constant  Value=2.0
  Constant_2.0_d6b90 : Constant  Value=2.0
  Constant_2.0_df382 : Constant  Value=2.0
  Constant_2.0_e9714 : Constant  Value=2.0
  Constant_99.502487562189_33882 : Constant  Value=99.502487562189
  Constant_99.502487562189_7f09e : Constant  Value=99.502487562189
  Constant_99.502487562189_b65d2 : Constant  Value=99.502487562189
  Constant_Ird_ref_96b7c : Constant  Value=Ird_ref
  Constant_Lm_pu_1c31e : Constant  Value=Lm_pu
  Constant_Lm_pu_396b7 : Constant  Value=Lm_pu
  Constant_Lm_pu_53d32 : Constant  Value=Lm_pu
  Constant_Lm_pu_af337 : Constant  Value=Lm_pu
  Constant_Lm_pu_af41f : Constant  Value=Lm_pu
  Constant_Lm_pu_ead88 : Constant  Value=Lm_pu
  Constant_Lm_pu_efc91 : Constant  Value=Lm_pu
  Constant_Rs_pu_c4346 : Constant  Value=Rs_pu
  Constant_Rs_pu_c9096 : Constant  Value=Rs_pu
  Constant_Sbase_1ce42 : Constant  Value=Sbase
  Constant_Sbase_51779 : Constant  Value=Sbase
  Constant_Sbase_6ba53 : Constant  Value=Sbase
  Constant_Sbase_83de6 : Constant  Value=Sbase
  Constant_Sbase_8d8d3 : Constant  Value=Sbase
  Constant_Sbase_95caa : Constant  Value=Sbase
  Constant_Sbase_9638e : Constant  Value=Sbase
  Constant_Sbase_9af04 : Constant  Value=Sbase
  Constant_Sbase_b33d3 : Constant  Value=Sbase
  Constant_Vbase_283f1 : Constant  Value=Vbase
  Constant_Vbase_329a9 : Constant  Value=Vbase
  Constant_Vbase_3f64c : Constant  Value=Vbase
  Constant_Vbase_63afa : Constant  Value=Vbase
  Constant_Vbase_71466 : Constant  Value=Vbase
  Constant_Vbase_8632b : Constant  Value=Vbase
  Constant_Vbase_96f25 : Constant  Value=Vbase
  Constant_Vbase_ae623 : Constant  Value=Vbase
  Constant_Vbase_fe687 : Constant  Value=Vbase
  Constant_f0_1f1e1 : Constant  Value=f0
  Constant_f0_6d4b4 : Constant  Value=f0
  Constant_f0_7398d : Constant  Value=f0
  Constant_f0_a0401 : Constant  Value=f0
  Constant_f0_c2c37 : Constant  Value=f0
  Constant_f0_ccbd8 : Constant  Value=f0
  Constant_f0_dcc55 : Constant  Value=f0
  Constant_f0_e60f8 : Constant  Value=f0
  Constant_f0_edad0 : Constant  Value=f0
  Constant_pi_250d6 : Constant  Value=pi
  Constant_pi_42664 : Constant  Value=pi
  Constant_pi_44b07 : Constant  Value=pi
  Constant_pi_502e5 : Constant  Value=pi
  Constant_pi_51bbd : Constant  Value=pi
  Constant_pi_7ca7d : Constant  Value=pi
  Constant_pi_b1ecf : Constant  Value=pi
  Constant_pi_ec6c6 : Constant  Value=pi
  Constant_pi_f8cb6 : Constant  Value=pi
  Divide_11b85 : Product  Inputs=*/
  Divide_1760f : Product  Inputs=*/
  Divide_278ad : Product  Inputs=*/
  Divide_4571a : Product  Inputs=*/
  Divide_791ea : Product  Inputs=*/
  Divide_a6066 : Product  Inputs=*/
  Divide_d910f : Product  Inputs=*/
  Divide_ded63 : Product  Inputs=*/
  Divide_fe07a : Product  Inputs=*/
  Power_36ccc : Math  Operator=pow
  Power_3f782 : Math  Operator=pow
  Power_545f8 : Math  Operator=pow
  Power_7f087 : Math  Operator=pow
  Power_9a329 : Math  Operator=pow
  Power_9f209 : Math  Operator=pow
  Power_9f395 : Math  Operator=pow
  Power_a1723 : Math  Operator=pow
  Power_c3737 : Math  Operator=pow
  Product_00437 : Product
  Product_01297 : Product
  Product_05e9f : Product
  Product_0b98c : Product
  Product_0cd14 : Product
  Product_0e61a : Product
  Product_0ed11 : Product
  Product_1120a : Product
  Product_12e61 : Product
  Product_1438d : Product
  Product_1924f : Product
  Product_1a316 : Product
  Product_215ee : Product
  Product_2562d : Product
  Product_33ba7 : Product
  Product_3bfef : Product
  Product_45037 : Product
  Product_480f9 : Product
  Product_4f068 : Product
  Product_55361 : Product
  Product_55b98 : Product
  Product_57a47 : Product
  Product_67b16 : Product
  Product_69e3c : Product
  Product_6ef27 : Product
  Product_75a56 : Product
  Product_7d8a0 : Product
  Product_7ea14 : Product
  Product_81d09 : Product
  Product_92e36 : Product
  Product_9b482 : Product
  Product_9eae5 : Product
  Product_aabb5 : Product
  Product_adc81 : Product
  Product_b3631 : Product
  Product_ba687 : Product
  Product_befe0 : Product
  Product_c98c1 : Product
  Product_cd052 : Product
  Product_cdabe : Product
  Product_d12aa : Product
  Product_d79df : Product
  Product_d9dca : Product
  Product_e6362 : Product
  Product_f572b : Product
  Product_f68b5 : Product
  Product_f78fb : Product
  Subtract_6399b : Sum  Inputs=+-
  Subtract_72085 : Sum  Inputs=+-
  Subtract_729ca : Sum  Inputs=+-
  Subtract_ca343 : Sum  Inputs=+-
  Subtract_f533b : Sum  Inputs=+-
  Subtract_fb3dc : Sum  Inputs=+-
  Blockout_d_Psi_dr_GFL_DFIG_7_75b07 : Outport
  wires:
  Constant_Lm_pu_efc91/1 -> Product_f572b/1
  Product_7d8a0/1 -> Divide_a6066/1
  Constant_2.0_63544/1 -> Power_545f8/2
  Constant_Sbase_6ba53/1 -> Divide_791ea/2
  Add_e290b/1 -> Blockout_d_Psi_dr_GFL_DFIG_7_75b07/1
  Constant_Vbase_3f64c/1 -> Power_c3737/1
  Subtract_ca343/1 -> Product_92e36/2
  Power_545f8/1 -> Product_0cd14/2
  State_Psi_ds_GFL_DFIG_7_652d4/1 -> Product_0b98c/2
  Product_92e36/1 -> Divide_ded63/1
  Product_81d09/1 -> Divide_278ad/1
  Constant_pi_f8cb6/1 -> Product_4f068/2
  Divide_4571a/1 -> Add_11a44/1
  Product_9eae5/1 -> Product_0b98c/1
  Constant_Lm_pu_af337/1 -> Product_ba687/2
  Constant_2.0_31ded/1 -> Power_9f395/2
  Product_01297/1 -> Divide_1760f/2
  Add_b780e/1 -> Product_7ea14/2
  Subtract_6399b/1 -> Product_1120a/2
  Product_4f068/1 -> Product_f68b5/1
  Product_0b98c/1 -> Product_480f9/1
  Product_d79df/1 -> Add_93a79/2
  State_Psi_dr_GFL_DFIG_7_ac80b/1 -> Product_f68b5/2
  Divide_791ea/1 -> Add_e290b/2
  Product_f78fb/1 -> Product_69e3c/1
  Constant_99.502487562189_b65d2/1 -> Product_9eae5/1
  Constant_pi_42664/1 -> Product_9eae5/2
  Product_adc81/1 -> Product_92e36/1
  Product_7ea14/1 -> Divide_791ea/1
  Power_7f087/1 -> Product_adc81/2
  Power_36ccc/1 -> Product_f572b/2
  Divide_11b85/1 -> Add_b780e/2
  Product_0cd14/1 -> Divide_11b85/2
  Constant_Vbase_ae623/1 -> Power_545f8/1
  Product_480f9/1 -> Product_1438d/1
  Constant_Lm_pu_ead88/1 -> Product_0cd14/1
  State_Psi_ds_GFL_DFIG_7_ccb41/1 -> Product_e6362/2
  Constant_Vbase_63afa/1 -> Power_36ccc/1
  Constant_-0.00995049504950496_e8382/1 -> Product_ba687/1
  Product_1438d/1 -> Divide_11b85/1
  Constant_100.497512437811_ea514/1 -> Product_3bfef/1
  Product_0e61a/1 -> Product_7ea14/1
  Constant_f0_c2c37/1 -> Product_81d09/2
  Constant_f0_dcc55/1 -> Product_1438d/2
  Constant_Vbase_8632b/1 -> Power_a1723/1
  Divide_ded63/1 -> Subtract_f533b/2
  Constant_Sbase_8d8d3/1 -> Product_480f9/2
  Product_f572b/1 -> Divide_fe07a/2
  Divide_d910f/1 -> Subtract_72085/2
  Product_1924f/1 -> Divide_d910f/1
  Constant_Vbase_96f25/1 -> Power_3f782/1
  Subtract_72085/1 -> Add_b780e/1
  Product_55b98/1 -> Product_67b16/1
  Subtract_f533b/1 -> Add_e290b/1
  Product_215ee/1 -> Divide_fe07a/1
  Power_a1723/1 -> Product_b3631/2
  Constant_100.497512437811_f5e6e/1 -> Product_4f068/1
  Constant_Sbase_9af04/1 -> Divide_ded63/2
  Product_d9dca/1 -> Divide_d910f/2
  Product_f68b5/1 -> Product_12e61/1
  Power_c3737/1 -> Product_d9dca/2
  Constant_Vbase_283f1/1 -> Power_7f087/1
  Constant_Ird_ref_96b7c/1 -> Subtract_72085/1
  Constant_Rs_pu_c4346/1 -> Product_75a56/2
  Constant_2.0_8a241/1 -> Power_c3737/2
  Constant_Lm_pu_af41f/1 -> Product_d9dca/1
  Product_75a56/1 -> Product_0e61a/1
  Constant_f0_a0401/1 -> Product_1924f/2
  Product_12e61/1 -> Product_1924f/1
  Constant_Sbase_83de6/1 -> Product_12e61/2
  Constant_2.0_df382/1 -> Power_9f209/2
  Constant_f0_ccbd8/1 -> Product_7d8a0/2
  Product_e6362/1 -> Product_57a47/1
  Power_9f209/1 -> Product_0e61a/2
  Constant_Vbase_fe687/1 -> Power_9f209/1
  Subtract_fb3dc/1 -> Product_cdabe/2
  Constant_1.1_42146/1 -> Product_75a56/1
  Constant_f0_7398d/1 -> Product_215ee/2
  Divide_fe07a/1 -> Subtract_ca343/2
  Constant_2.0_b3930/1 -> Power_36ccc/2
  Product_57a47/1 -> Product_215ee/1
  Constant_Sbase_51779/1 -> Product_57a47/2
  Product_befe0/1 -> Product_e6362/1
  Constant_pi_502e5/1 -> Product_befe0/2
  Constant_99.502487562189_33882/1 -> Product_befe0/1
  Divide_a6066/1 -> Subtract_ca343/1
  Product_55361/1 -> Divide_a6066/2
  Power_3f782/1 -> Product_55361/2
  Constant_2.0_e9714/1 -> Power_3f782/2
  Constant_Lm_pu_1c31e/1 -> Product_55361/1
  Product_c98c1/1 -> Product_7d8a0/1
  Constant_Sbase_1ce42/1 -> Product_c98c1/2
  Product_0ed11/1 -> Product_c98c1/1
  State_Psi_dr_GFL_DFIG_7_f20f7/1 -> Product_0ed11/2
  Product_3bfef/1 -> Product_0ed11/1
  Product_00437/1 -> Product_aabb5/1
  Constant_pi_44b07/1 -> Product_3bfef/2
  Constant_2.0_76225/1 -> Power_7f087/2
  Product_d12aa/1 -> Product_adc81/1
  Constant_Rs_pu_c9096/1 -> Product_d12aa/2
  State_w_m_GFL_DFIG_7_c0fab/1 -> Subtract_729ca/2
  Constant_1.1_4732a/1 -> Product_d12aa/1
  Add_93a79/1 -> Subtract_f533b/1
  Subtract_729ca/1 -> Product_d79df/2
  Product_67b16/1 -> Subtract_729ca/1
  Constant_f0_6d4b4/1 -> Product_67b16/2
  Constant_pi_51bbd/1 -> Product_55b98/2
  Constant_2.0_4f40a/1 -> Product_55b98/1
  State_Psi_qr_GFL_DFIG_7_8feb7/1 -> Product_d79df/1
  Add_11a44/1 -> Add_93a79/1
  State_Phi_ra_GFL_DFIG_7_e382b/1 -> Add_11a44/2
  Product_69e3c/1 -> Divide_4571a/2
  Constant_f0_edad0/1 -> Product_69e3c/2
  Constant_Sbase_b33d3/1 -> Product_f78fb/2
  Product_9b482/1 -> Product_00437/1
  Constant_pi_7ca7d/1 -> Product_f78fb/1
  Product_1120a/1 -> Divide_4571a/1
  Divide_278ad/1 -> Subtract_6399b/2
  Product_b3631/1 -> Divide_278ad/2
  Constant_2.0_74f55/1 -> Power_a1723/2
  Constant_Lm_pu_396b7/1 -> Product_b3631/1
  Product_aabb5/1 -> Product_81d09/1
  Constant_Sbase_95caa/1 -> Product_aabb5/2
  State_Psi_qs_GFL_DFIG_7_a7547/1 -> Product_00437/2
  Constant_pi_b1ecf/1 -> Product_9b482/2
  Constant_99.502487562189_7f09e/1 -> Product_9b482/1
  Divide_1760f/1 -> Subtract_6399b/1
  Power_9a329/1 -> Product_01297/2
  Constant_2.0_480a2/1 -> Power_9a329/2
  Product_2562d/1 -> Divide_1760f/1
  Constant_Vbase_71466/1 -> Power_9a329/1
  Product_45037/1 -> Product_cdabe/1
  Constant_Lm_pu_53d32/1 -> Product_01297/1
  Constant_2.0_d6b90/1 -> Product_33ba7/1
  Constant_f0_1f1e1/1 -> Product_2562d/2
  Product_05e9f/1 -> Product_2562d/1
  Constant_Sbase_9638e/1 -> Product_05e9f/2
  Product_1a316/1 -> Product_05e9f/1
  State_Psi_qr_GFL_DFIG_7_b0873/1 -> Product_1a316/2
  Product_6ef27/1 -> Product_1a316/1
  Constant_pi_ec6c6/1 -> Product_6ef27/2
  Constant_100.497512437811_62b2c/1 -> Product_6ef27/1
  Product_cdabe/1 -> Product_1120a/1
  State_w_m_GFL_DFIG_7_ede24/1 -> Subtract_fb3dc/2
  Product_cd052/1 -> Subtract_fb3dc/1
  Constant_f0_e60f8/1 -> Product_cd052/2
  Product_33ba7/1 -> Product_cd052/1
  Constant_pi_250d6/1 -> Product_33ba7/2
  Power_9f395/1 -> Product_45037/2
  Constant_Vbase_329a9/1 -> Power_9f395/1
  Product_ba687/1 -> Product_45037/1

== system IEEE30_case/GFL_DFIG_7/d_Psi_ds_GFL_DFIG_7_block ==
  note: d_Psi_ds_GFL_DFIG_7 in IEEE30_case
      | $2\,\pi \,\Psi _{\mathrm{qs},\mathrm{GFL},\mathrm{DFIG},7}\,f_{0}-\mathrm{Vbase}\,\left(v_{d,\mathrm{GFL},\mathrm{DFIG},7}\,\cos\left(\theta _{\mathrm{pllr},\mathrm{GFL},\mathrm{DFIG},7}\right)-v_{q,\mathrm{GFL},\mathrm{DFIG},7}\,\sin\left(\theta _{\mathrm{pllr},\mathrm{GFL},\mathrm{DFIG},7}\right)\right)+\frac{\mathrm{Rs}_{\mathrm{pu}}\,{\mathrm{Vbase}}^2\,\left(\frac{99.502487562189\,\pi \,\Psi _{\mathrm{dr},\mathrm{GFL},\mathrm{DFIG},7}\,\mathrm{Sbase}\,f_{0}}{\mathrm{Lm}_{\mathrm{pu}}\,{\mathrm{Vbase}}^2}-\frac{100.497512437811\,\pi \,\Psi _{\mathrm{ds},\mathrm{GFL},\mathrm{DFIG},7}\,\mathrm{Sbase}\,f_{0}}{\mathrm{Lm}_{\mathrm{pu}}\,{\mathrm{Vbase}}^2}\right)}{\mathrm{Sbase}}$
      | Automatically generated on 2025-11-01 18:32:31 .
  State_Psi_qs_GFL_DFIG_7_b4caa : Inport
  State_Psi_dr_GFL_DFIG_7_0949a : Inport  Port=2
  State_Psi_ds_GFL_DFIG_7_d7878 : Inport  Port=3
  Input_v_d_GFL_DFIG_7_61464 : Inport  Port=4
  State_theta_pllr_GFL_DFIG_7_d96f9 : Inport  Port=5
  Input_v_q_GFL_DFIG_7_712eb : Inport  Port=6
  State_theta_pllr_GFL_DFIG_7_2fe4a : Inport  Port=7
  Add_14c1b : Sum
  Add_1e3db : Sum
  Add_82052 : Sum
  Constant_-1_59c85 : Constant  Value=-1
  Constant_-99.502487562189_d02e9 : Constant  Value=-99.502487562189
  Constant_100.497512437811_15211 : Constant  Value=100.497512437811
  Constant_2.0_24635 : Constant  Value=2.0
  Constant_2.0_8d08e : Constant  Value=2.0
  Constant_2.0_d3c3c : Constant  Value=2.0
  Constant_2.0_fef91 : Constant  Value=2.0
  Constant_Lm_pu_3c8a2 : Constant  Value=Lm_pu
  Constant_Lm_pu_42e06 : Constant  Value=Lm_pu
  Constant_Rs_pu_091bc : Constant  Value=Rs_pu
  Constant_Sbase_5a8e9 : Constant  Value=Sbase
  Constant_Sbase_8340d : Constant  Value=Sbase
  Constant_Sbase_f5d7c : Constant  Value=Sbase
  Constant_Vbase_35267 : Constant  Value=Vbase
  Constant_Vbase_8adcd : Constant  Value=Vbase
  Constant_Vbase_9aef6 : Constant  Value=Vbase
  Constant_Vbase_b591a : Constant  Value=Vbase
  Constant_f0_05f5c : Constant  Value=f0
  Constant_f0_54161 : Constant  Value=f0
  Constant_f0_6b606 : Constant  Value=f0
  Constant_pi_338cc : Constant  Value=pi
  Constant_pi_56050 : Constant  Value=pi
  Constant_pi_6cd23 : Constant  Value=pi
  Divide_54757 : Product  Inputs=*/
  Divide_89b73 : Product  Inputs=*/
  Divide_c20b8 : Product  Inputs=*/
  MathFunc_cos_7fee8 : Trigonometry  Operator=cos
  MathFunc_sin_b369d : Trigonometry
  Power_1a83a : Math  Operator=pow
  Power_9e51d : Math  Operator=pow
  Power_ee1cb : Math  Operator=pow
  Product_019c6 : Product
  Product_01ae1 : Product
  Product_129e7 : Product
  Product_24dc0 : Product
  Product_{30489,36677,66212,74955} (4 alike) : Product
  Product_3b5bb : Product
  Product_590df : Product
  Product_5955b : Product
  Product_64b35 : Product
  Product_70d4a : Product
  Product_74c0e : Product
  Product_7a9a7 : Product
  Product_95b51 : Product
  Product_9ca6e : Product
  Product_a60f9 : Product
  Product_c012f : Product
  Subtract_c13d5 : Sum  Inputs=+-
  Blockout_d_Psi_ds_GFL_DFIG_7_0935c : Outport
  wires:
  Constant_100.497512437811_15211/1 -> Product_590df/1
  Constant_-99.502487562189_d02e9/1 -> Product_66212/1
  Product_9ca6e/1 -> Add_82052/2
  Constant_pi_56050/1 -> Product_66212/2
  Product_66212/1 -> Product_64b35/1
  Constant_pi_338cc/1 -> Product_590df/2
  Divide_54757/1 -> Add_1e3db/2
  State_Psi_dr_GFL_DFIG_7_0949a/1 -> Product_64b35/2
  Input_v_q_GFL_DFIG_7_712eb/1 -> Product_3b5bb/1
  Product_019c6/1 -> Divide_54757/1
  State_Psi_ds_GFL_DFIG_7_d7878/1 -> Product_70d4a/2
  Constant_f0_6b606/1 -> Product_019c6/2
  Product_590df/1 -> Product_70d4a/1
  Product_64b35/1 -> Product_5955b/1
  Constant_Rs_pu_091bc/1 -> Product_129e7/1
  Constant_Sbase_f5d7c/1 -> Product_5955b/2
  Product_74955/1 -> Divide_89b73/1
  Constant_-1_59c85/1 -> Product_a60f9/1
  Constant_Vbase_9aef6/1 -> Power_1a83a/1
  Constant_2.0_24635/1 -> Power_ee1cb/2
  Constant_2.0_d3c3c/1 -> Power_1a83a/2
  Divide_89b73/1 -> Subtract_c13d5/2
  Product_70d4a/1 -> Product_c012f/1
  Constant_Sbase_8340d/1 -> Product_c012f/2
  Constant_pi_6cd23/1 -> Product_01ae1/2
  Constant_Vbase_8adcd/1 -> Power_ee1cb/1
  Power_ee1cb/1 -> Product_95b51/2
  Product_5955b/1 -> Product_24dc0/1
  Constant_f0_54161/1 -> Product_24dc0/2
  Constant_Lm_pu_42e06/1 -> Product_36677/1
  Product_3b5bb/1 -> Add_14c1b/2
  Power_1a83a/1 -> Product_36677/2
  Product_c012f/1 -> Product_019c6/1
  Product_01ae1/1 -> Product_74c0e/1
  Constant_Lm_pu_3c8a2/1 -> Product_95b51/1
  Constant_Vbase_b591a/1 -> Power_9e51d/1
  Product_30489/1 -> Subtract_c13d5/1
  Constant_2.0_fef91/1 -> Power_9e51d/2
  Product_24dc0/1 -> Divide_c20b8/1
  Product_36677/1 -> Divide_c20b8/2
  Product_95b51/1 -> Divide_54757/2
  Constant_2.0_8d08e/1 -> Product_01ae1/1
  MathFunc_cos_7fee8/1 -> Product_7a9a7/2
  Power_9e51d/1 -> Product_129e7/2
  State_Psi_qs_GFL_DFIG_7_b4caa/1 -> Product_74c0e/2
  Divide_c20b8/1 -> Add_1e3db/1
  State_theta_pllr_GFL_DFIG_7_d96f9/1 -> MathFunc_cos_7fee8/1
  Input_v_d_GFL_DFIG_7_61464/1 -> Product_a60f9/2
  State_theta_pllr_GFL_DFIG_7_2fe4a/1 -> MathFunc_sin_b369d/1
  Product_129e7/1 -> Product_74955/1
  Product_a60f9/1 -> Product_7a9a7/1
  Add_1e3db/1 -> Product_74955/2
  MathFunc_sin_b369d/1 -> Product_3b5bb/2
  Product_74c0e/1 -> Product_30489/1
  Constant_Sbase_5a8e9/1 -> Divide_89b73/2
  Constant_f0_05f5c/1 -> Product_30489/2
  Product_7a9a7/1 -> Add_14c1b/1
  Add_82052/1 -> Blockout_d_Psi_ds_GFL_DFIG_7_0935c/1
  Constant_Vbase_35267/1 -> Product_9ca6e/1
  Add_14c1b/1 -> Product_9ca6e/2
  Subtract_c13d5/1 -> Add_82052/1
